simulink library "sensors_lib"  (R2016b)
settings: Solver=ode45  StartTime=0.0  StopTime=10.0  RelTol=1e-3  EnableMultiTasking=on
undefined symbols (not defined in the file or in its folder): mag_vec_body_T, meas_deg_err, omega_body_radps_gyro, sun_vec_body_sunsensor
libraries: bus_stubs_template x1, gyroscope_lib x1, magnetometer_lib x1, sun_sensor_lib x1
settings Model: Creator=bbarz_000  LastModifiedBy=Taylor
settings DataIOCC: LimitDataPoints=on
settings OptimizationCC: LifeSpan=inf
settings DebuggingCC: AllowSymbolicDim=off  SFUnexpectedBacktrackingDiag=warning  SFNoUnconditionalDefaultTransitionDiag=warning  SFExecutionAtInitializationDiag=none
settings GRTTargetCC: TargetLangStandard=C89/C90 (ANSI)  GeneratePreprocessorConditionals=Disable all
settings ConfigComp: CovMetricSettings=dw  CovHtmlReporting=on  CovSaveCumulativeToWorkspaceVar=on  CovSaveSingleToWorkspaceVar=on  CovExternalEMLEnable=off

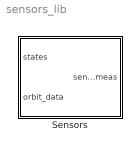
== system sensors_lib ==
  Sensors : Subsystem

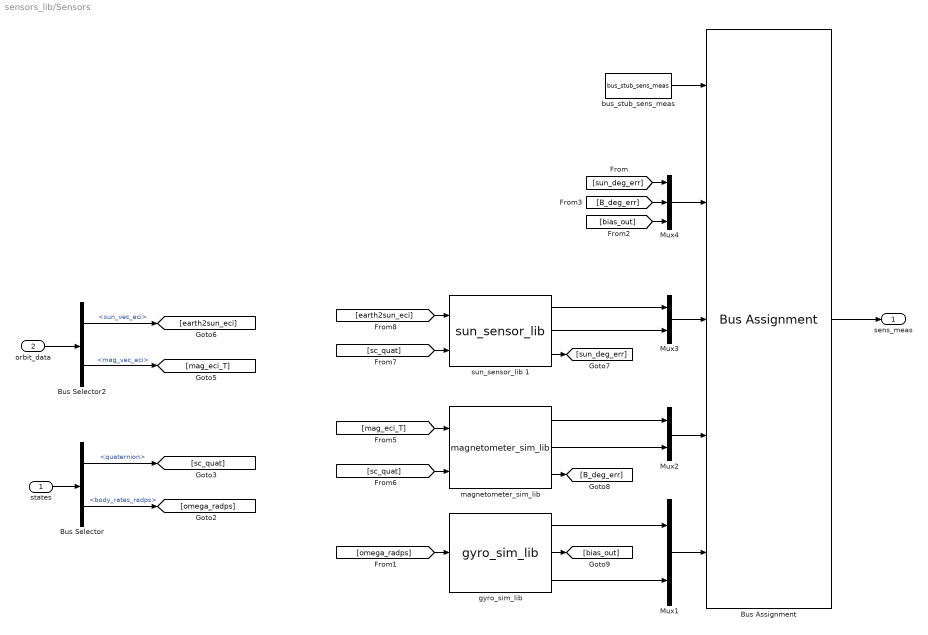
== system sensors_lib/Sensors ==
  states : Inport  OutDataTypeStr=Bus: states
  orbit_data : Inport  Port=2  OutDataTypeStr=Bus: orbit_data
  Bus Assignment : BusAssignment  AssignedSignals=meas_deg_err,sun_vec_body_sunsensor,mag_vec_body_T,omega_body_radps_gyro
  Bus Selector : BusSelector  OutputSignals=quaternion,body_rates_radps
  Bus Selector2 : BusSelector  OutputSignals=sun_vec_eci,mag_vec_eci
  Mux1 : Mux  Inputs=[3 1]
  Mux2 : Mux  Inputs=[3 1]
  Mux3 : Mux  Inputs=[3 1]
  Mux4 : Mux  Inputs=[1 1 3]
  bus_stub_sens_meas : bus_stubs_template/bus_stub_sens_meas
  gyro_sim_lib : gyroscope_lib/gyro_sim_lib
  magnetometer_sim_lib : magnetometer_lib/magnetometer_sim_lib
  sun_sensor_lib 1 : sun_sensor_lib/sun_sensor_lib 
  sens_meas : Outport
  wires:
  states/1 -> Bus Selector/1
  Bus Assignment/1 -> sens_meas/1
  bus_stub_sens_meas/1 -> Bus Assignment/1
  orbit_data/1 -> Bus Selector2/1
  gyro_sim_lib/1 -> Mux1/1
  gyro_sim_lib/3 -> Mux1/2
  magnetometer_sim_lib/1 -> Mux2/1
  magnetometer_sim_lib/2 -> Mux2/2
  sun_sensor_lib 1/1 -> Mux3/1
  sun_sensor_lib 1/2 -> Mux3/2
  Mux4/1 -> Bus Assignment/2
  Mux1/1 -> Bus Assignment/5
  Bus Selector/2 -> [omega_radps]  "<body_rates_radps>"
  Bus Selector/1 -> [sc_quat]  "<quaternion>"
  Bus Selector2/2 -> [mag_eci_T]  "<mag_vec_eci>"
  Bus Selector2/1 -> [earth2sun_eci]  "<sun_vec_eci>"
  [omega_radps] -> gyro_sim_lib/1
  [mag_eci_T] -> magnetometer_sim_lib/1
  [sc_quat] -> magnetometer_sim_lib/2
  [sc_quat] -> sun_sensor_lib 1/2
  [earth2sun_eci] -> sun_sensor_lib 1/1
  Mux3/1 -> Bus Assignment/3
  Mux2/1 -> Bus Assignment/4
  sun_sensor_lib 1/3 -> [sun_deg_err]
  [sun_deg_err] -> Mux4/1
  gyro_sim_lib/2 -> [bias_out]
  [bias_out] -> Mux4/3
  magnetometer_sim_lib/3 -> [B_deg_err]
  [B_deg_err] -> Mux4/2
